simulink model "simlab1a"  (R2021a)
settings: Solver=ode4  StartTime=0.0  StopTime=10.0  FixedStep=0.001  RelTol=1e-3
settings Model: Creator=martinsundar  LastModifiedBy=martinsundar

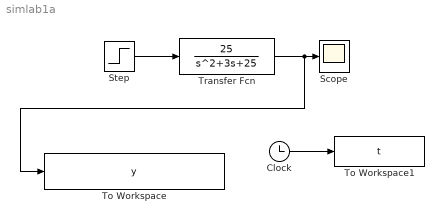
== system simlab1a ==
  Clock : Clock
  Scope : Scope
  Step : Step  After=10  SampleTime=0
  To Workspace : ToWorkspace  VariableName=y  SampleTime=-1
  To Workspace1 : ToWorkspace  VariableName=t  SampleTime=-1
  Transfer Fcn : TransferFcn  Numerator=[25]  Denominator=[1 3 25]
  wires:
  Step/1 -> Transfer Fcn/1
  Transfer Fcn/1 -> To Workspace/1, Scope/1
  Clock/1 -> To Workspace1/1
